simulink model "SuspensionModel"  (R2020b)
settings: Solver=VariableStepAuto  StartTime=0.0  StopTime=100  MaxStep=0.001  RelTol=1e-3
settings Model: Creator=BIDITA PAUL  LastModifiedBy=BIDITA PAUL

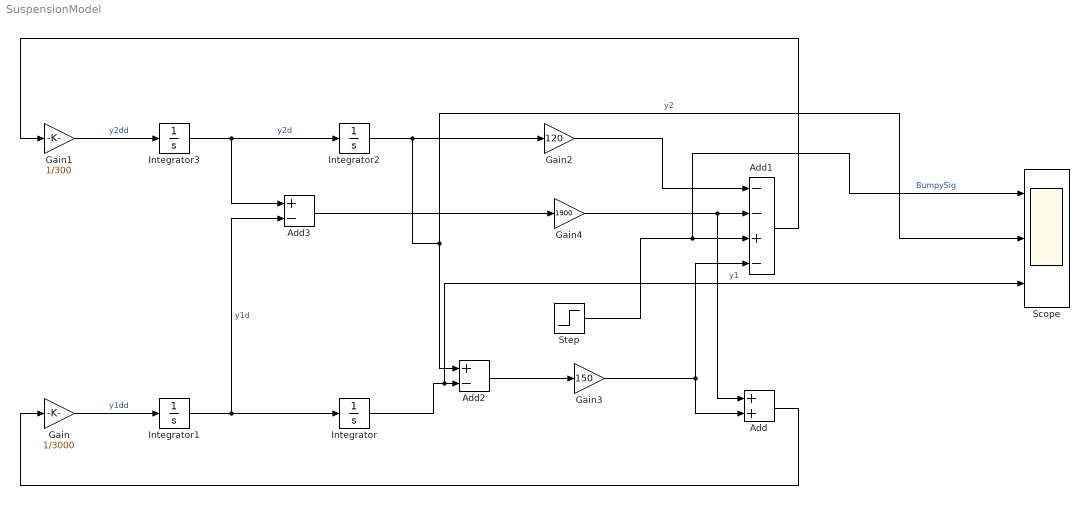
== system SuspensionModel ==
  Add : Sum
  Add1 : Sum  Inputs=--+-
  Add2 : Sum  Inputs=+-
  Add3 : Sum  Inputs=+-
  Gain : Gain  Gain=1/3000
  Gain1 : Gain  Gain=1/300
  Gain2 : Gain  Gain=120
  Gain3 : Gain  Gain=150
  Gain4 : Gain  Gain=1900
  Integrator{,1..3} (4 alike) : Integrator
  Scope : Scope  NumInputPorts=3
  Step : Step  Time=10  SampleTime=0
  wires:
  Integrator1/1 -> Add3/2, Integrator/1  "y1d"
  Integrator3/1 -> Add3/1, Integrator2/1  "y2d"
  Add3/1 -> Gain4/1
  Integrator2/1 -> Gain2/1, Scope/2, Add2/1  "y2"
  Integrator/1 -> Scope/3, Add2/2  "y1"
  Add2/1 -> Gain3/1
  Gain/1 -> Integrator1/1  "y1dd"
  Gain1/1 -> Integrator3/1  "y2dd"
  Add1/1 -> Gain1/1
  Add/1 -> Gain/1
  Gain3/1 -> Add1/4, Add/2
  Gain4/1 -> Add/1, Add1/2
  Gain2/1 -> Add1/1
  Step/1 -> Add1/3, Scope/1  "BumpySig"
